simulink model "ABS_MP_TS9"  (Simulink 7.6)
settings: Solver=ode45  SolverMode=SingleTasking  StartTime=0  StopTime=12  FixedStep=0.002  RelTol=1e-3  AbsTol=1e-6
libraries: Solver_SF x1
settings Model: Creator=bduprey  LastModifiedBy=hkawanishi  ExtModeTrigMode=oneshot  ExtModeArmWhenConnect=off
settings DataIOCC: LimitDataPoints=off
settings OptimizationCC: BlockReduction=off  BooleanDataType=off
settings DebuggingCC: SaveWithParameterizedLinksMsg=none  SignalResolutionControl=TryResolveAllWithWarning  SolverPrmCheckMsg=none  MultiTaskDSMMsg=warning  MultiTaskCondExecSysMsg=none  StrictBusMsg=None
settings HardwareCC: TargetUnknown=on
settings RTWCC: TemplateMakefile=grt_vc.tmf  IncludeERTFirstTime=on
settings GRTTargetCC: TargetFcnLib=ansi_tfl_tmw.mat

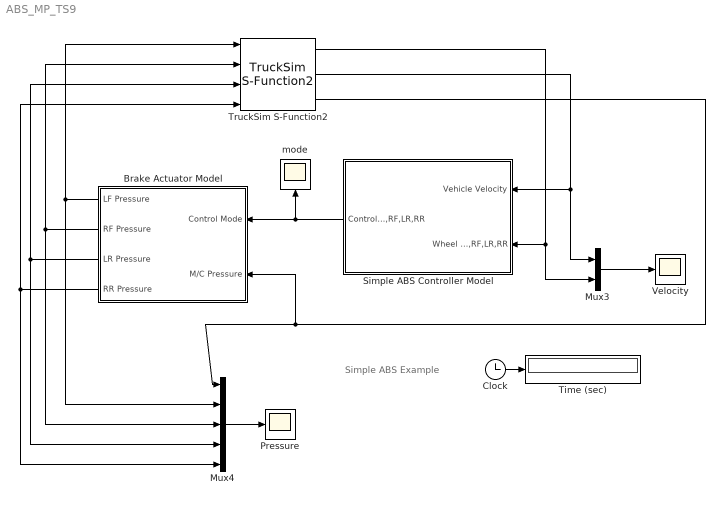
== system ABS_MP_TS9 ==
  note: Simple ABS Example
  Brake Actuator Model : Subsystem
  Clock : Clock
      settings: Decimation=10
  Mux3 : Mux  Inputs=2
  Mux4 : Mux  Inputs=5
  Pressure : Scope
      settings: TickLabels=on  YMin=0  YMax=10  DataFormat=Array  SampleTime=100
  Simple ABS Controller Model : Subsystem
  Time (sec) : Display
      settings: Format=bank  Decimation=100
  TruckSim S-Function2 : Solver_SF/TruckSim S-Function2  Priority=1  SIMFILE=simfile.sim
  Velocity : Scope
      settings: TickLabels=on  YMin=-10  YMax=100  DataFormat=Array  SampleTime=100
  mode : Scope
      settings: TickLabels=on  YMin=0  YMax=1  DataFormat=Array  SampleTime=100
  wires:
  Mux4/1 -> Pressure/1
  TruckSim S-Function2/2 -> Mux3/1, Simple ABS Controller Model/1(Vehicle Velocity)
  TruckSim S-Function2/1 -> Mux3/2, Simple ABS Controller Model/2(Wheel Velocity LF,RF,LR,RR)
  Clock/1 -> Time (sec)/1
  Simple ABS Controller Model/1(Control Mode LF,RF,LR,RR) -> Brake Actuator Model/1(Control Mode), mode/1
  Mux3/1 -> Velocity/1
  TruckSim S-Function2/3 -> Mux4/1, Brake Actuator Model/2(M/C Pressure)
  Brake Actuator Model/4(RR Pressure) -> Mux4/5, TruckSim S-Function2/4
  Brake Actuator Model/3(LR Pressure) -> Mux4/4, TruckSim S-Function2/3
  Brake Actuator Model/2(RF Pressure) -> Mux4/3, TruckSim S-Function2/2
  Brake Actuator Model/1(LF Pressure) -> Mux4/2, TruckSim S-Function2/1

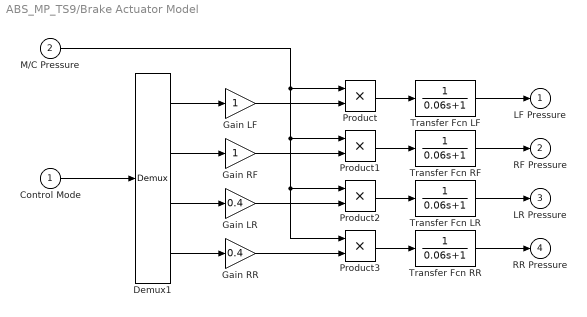
== system ABS_MP_TS9/Brake Actuator Model ==
  Control Mode : Inport
  M/C Pressure : Inport  Port=2
  Demux1 : Demux
  Gain LF : Gain  SaturateOnIntegerOverflow=on  OutDataTypeStr=Inherit: Same as input  ParamDataTypeStr=Inherit: Same as input
  Gain LR : Gain  Gain=0.4  SaturateOnIntegerOverflow=on  OutDataTypeStr=Inherit: Same as input  ParamDataTypeStr=Inherit: Same as input
  Gain RF : Gain  SaturateOnIntegerOverflow=on  OutDataTypeStr=Inherit: Same as input  ParamDataTypeStr=Inherit: Same as input
  Gain RR : Gain  Gain=0.4  SaturateOnIntegerOverflow=on  OutDataTypeStr=Inherit: Same as input  ParamDataTypeStr=Inherit: Same as input
  Product{,1..3} (4 alike) : Product  SaturateOnIntegerOverflow=on  RndMeth=Zero  InputSameDT=on  OutDataTypeStr=Inherit: Same as first input
  Transfer Fcn LF : TransferFcn  Denominator=[0.06 1]
  Transfer Fcn LR : TransferFcn  Denominator=[0.06 1]
  Transfer Fcn RF : TransferFcn  Denominator=[0.06 1]
  Transfer Fcn RR : TransferFcn  Denominator=[0.06 1]
  LF Pressure : Outport  InitialOutput=0
  RF Pressure : Outport  Port=2  InitialOutput=0
  LR Pressure : Outport  Port=3  InitialOutput=0
  RR Pressure : Outport  Port=4  InitialOutput=0
  wires:
  Control Mode/1 -> Demux1/1
  Gain LF/1 -> Product/2
  Gain RF/1 -> Product1/2
  Gain LR/1 -> Product2/2
  Gain RR/1 -> Product3/2
  M/C Pressure/1 -> Product/1, Product1/1, Product2/1, Product3/1
  Product/1 -> Transfer Fcn LF/1
  Transfer Fcn LF/1 -> LF Pressure/1
  Product1/1 -> Transfer Fcn RF/1
  Product2/1 -> Transfer Fcn LR/1
  Product3/1 -> Transfer Fcn RR/1
  Demux1/1 -> Gain LF/1
  Demux1/2 -> Gain RF/1
  Demux1/3 -> Gain LR/1
  Demux1/4 -> Gain RR/1
  Transfer Fcn RF/1 -> RF Pressure/1
  Transfer Fcn LR/1 -> LR Pressure/1
  Transfer Fcn RR/1 -> RR Pressure/1

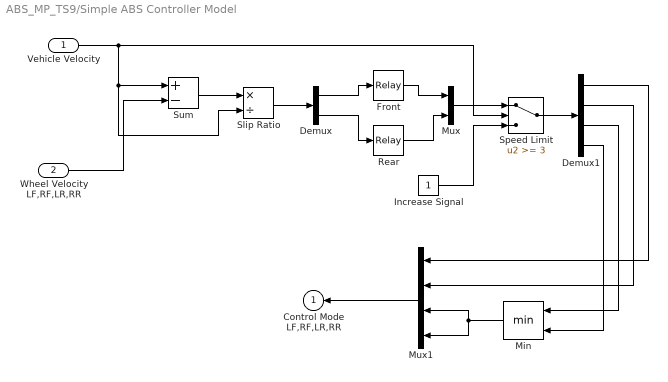
== system ABS_MP_TS9/Simple ABS Controller Model ==
  Vehicle Velocity : Inport
  Wheel Velocity LF,RF,LR,RR : Inport  Port=2
  Demux : Demux  Outputs=[2 2]
  Demux1 : Demux
  Front : Relay  OnSwitchValue=0.1  OffSwitchValue=0.05  OnOutputValue=0  OffOutputValue=1
  Increase Signal : Constant
  Min : MinMax  Inputs=2  SaturateOnIntegerOverflow=on  InputSameDT=on
  Mux : Mux  Inputs=2
  Mux1 : Mux
  Rear : Relay  OnSwitchValue=0.1  OffSwitchValue=0.05  OnOutputValue=0  OffOutputValue=1
  Slip Ratio : Product  Inputs=*/  SaturateOnIntegerOverflow=on  RndMeth=Zero  InputSameDT=on  OutDataTypeStr=Inherit: Same as first input
  Speed Limit : Switch  Threshold=3  SaturateOnIntegerOverflow=on  InputSameDT=on
  Sum : Sum  Inputs=+-  SaturateOnIntegerOverflow=on  InputSameDT=on  OutDataTypeStr=Inherit: Same as first input
  Control Mode LF,RF,LR,RR : Outport  InitialOutput=0
  wires:
  Vehicle Velocity/1 -> Sum/1, Slip Ratio/2, Speed Limit/2
  Speed Limit/1 -> Demux1/1
  Increase Signal/1 -> Speed Limit/3
  Sum/1 -> Slip Ratio/1
  Slip Ratio/1 -> Demux/1
  Mux/1 -> Speed Limit/1
  Min/1 -> Mux1/3, Mux1/4
  Demux1/3 -> Min/1
  Demux1/4 -> Min/2
  Demux1/2 -> Mux1/2
  Demux1/1 -> Mux1/1
  Mux1/1 -> Control Mode LF,RF,LR,RR/1
  Front/1 -> Mux/1
  Demux/1 -> Front/1
  Demux/2 -> Rear/1
  Rear/1 -> Mux/2
  Wheel Velocity LF,RF,LR,RR/1 -> Sum/2
